simulink model "extended_estimator"  (R2022b)
settings: Solver=FixedStepAuto  StartTime=0.0  StopTime=30  FixedStep=0.001  RelTol=1e-3
values from neighbouring files (symbols this model uses):
  A = -3    [para.m]
  As = [0 1 0;-omega^2 0 0; 1 0 -3]    [para.m]
  B = 1    [para.m]
  Bs = [0 ; 0 ;1]    [para.m]
  C = 1    [para.m]
  Cs = [0 0 1]    [para.m]
  D = 0    [para.m]
  Ds = 0    [para.m]
  K = place(A,B,-5)    [para.m]
  L = place(As',Cs',[-19 -20 -21])'    [para.m]
  omega = 10    [para.m]
settings Model: Creator=mxiaoxin  LastModifiedBy=mxiaoxin

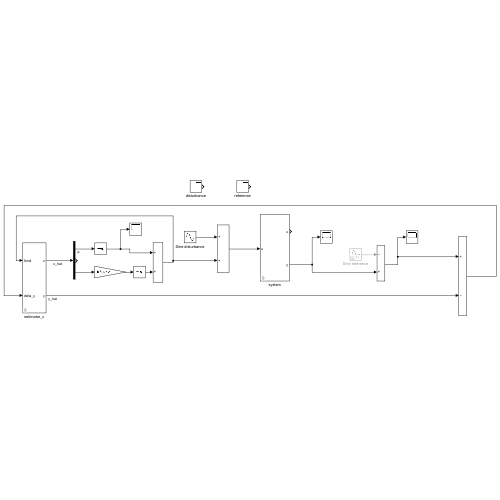
[thumbnail: Simulink's stored preview of the top-level diagram]
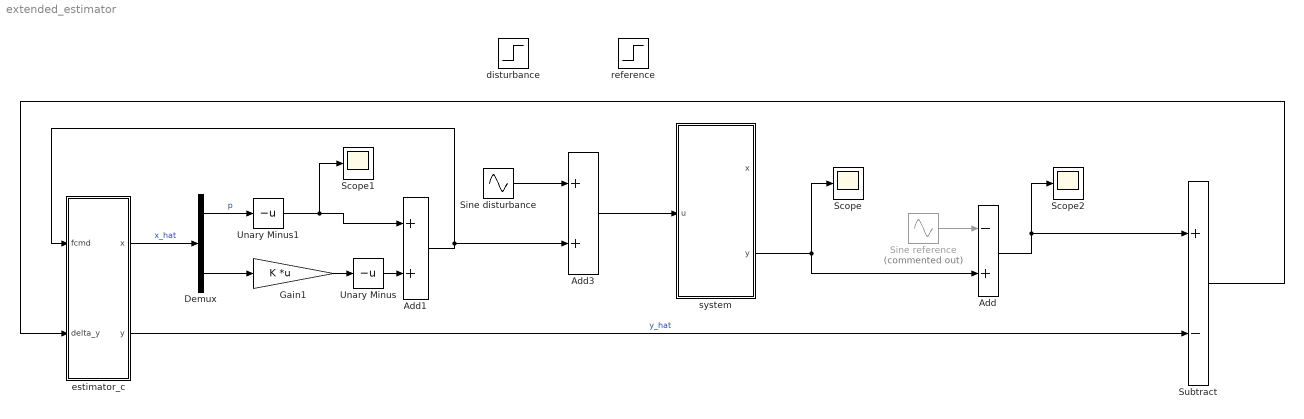
== system extended_estimator ==
  Add : Sum  Inputs=-+
  Add1 : Sum
  Add3 : Sum
  Demux : Demux  Outputs=3
  Gain1 : Gain  Gain=K  Multiplication=Matrix(K*u) (u vector)
  Scope : Scope
  Scope1 : Scope
  Scope2 : Scope
  Sine disturbance : Sin  Frequency=omega  Phase=180  SampleTime=0
  Sine reference : Sin  Commented=on  Frequency=omega  SampleTime=0
  Subtract : Sum  Inputs=+-
  Unary Minus : UnaryMinus
  Unary Minus1 : UnaryMinus
  disturbance : Step  SampleTime=0
  estimator_c : Subsystem  mask{x_A=As, x_B=Bs, x_C=Cs, x_D=Ds, xl=L}
      mask prompts: x_A "A"; x_B "B"; x_C "C"; x_D "D"; xl "L"
      mask DialogControl ParameterGroupVar Prompt: 系统
      mask DialogControl Container3 Prompt: feedback
  reference : Step  Time=0  SampleTime=0
  system : Subsystem  mask{Ac=A, Bc=B, Cc=C, Dc=D, x_0=0}
      mask DialogControl ParameterGroupVar Prompt: 参数
  wires:
  Subtract/1 -> estimator_c/2(delta_y)
  estimator_c/1(x) -> Demux/1  "x_hat"
  Unary Minus1/1 -> Add1/1, Scope1/1
  Gain1/1 -> Unary Minus/1
  Unary Minus/1 -> Add1/2
  Demux/1 -> Unary Minus1/1  "p"
  system/2(y) -> Add/2, Scope/1
  Add1/1 -> Add3/2, estimator_c/1(fcmd)
  Add3/1 -> system/1(u)
  estimator_c/2(y) -> Subtract/2  "y_hat"
  Sine disturbance/1 -> Add3/1
  Demux/3 -> Gain1/1
  Add/1 -> Subtract/1, Scope2/1
  Sine reference/1 -> Add/1

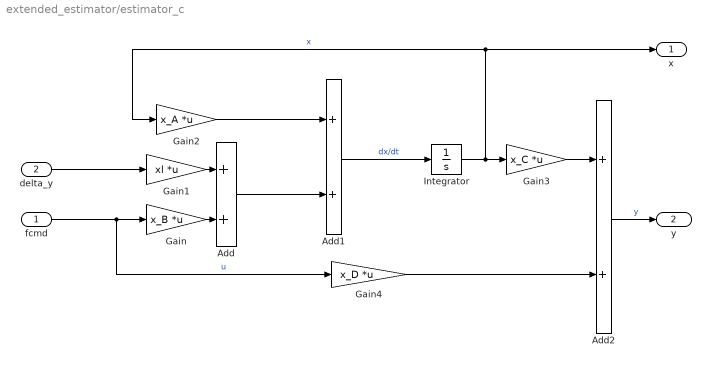
== system extended_estimator/estimator_c ==
  fcmd : Inport
  delta_y : Inport  Port=2
  Add : Sum
  Add1 : Sum
  Add2 : Sum
  Gain : Gain  Gain=x_B  Multiplication=Matrix(K*u)
  Gain1 : Gain  Gain=xl  Multiplication=Matrix(K*u)
  Gain2 : Gain  Gain=x_A  Multiplication=Matrix(K*u)
  Gain3 : Gain  Gain=x_C  Multiplication=Matrix(K*u)
  Gain4 : Gain  Gain=x_D  Multiplication=Matrix(K*u)
  Integrator : Integrator
  x : Outport
  y : Outport  Port=2
  wires:
  Gain2/1 -> Add1/1
  Add/1 -> Add1/2
  Add1/1 -> Integrator/1  "dx/dt"
  Integrator/1 -> Gain3/1, x/1, Gain2/1  "x"
  Gain1/1 -> Add/1
  delta_y/1 -> Gain1/1
  fcmd/1 -> Gain/1, Gain4/1  "u"
  Gain/1 -> Add/2
  Gain3/1 -> Add2/1
  Gain4/1 -> Add2/2
  Add2/1 -> y/1  "y"

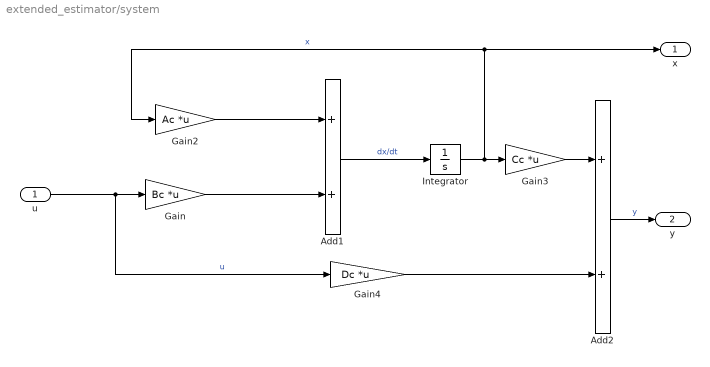
== system extended_estimator/system ==
  u : Inport
  Add1 : Sum
  Add2 : Sum
  Gain : Gain  Gain=Bc  Multiplication=Matrix(K*u)
  Gain2 : Gain  Gain=Ac  Multiplication=Matrix(K*u)
  Gain3 : Gain  Gain=Cc  Multiplication=Matrix(K*u)
  Gain4 : Gain  Gain=Dc  Multiplication=Matrix(K*u)
  Integrator : Integrator  InitialCondition=x_0
  x : Outport
  y : Outport  Port=2
  wires:
  Gain2/1 -> Add1/1
  Gain/1 -> Add1/2
  Add1/1 -> Integrator/1  "dx/dt"
  Integrator/1 -> Gain3/1, Gain2/1, x/1  "x"
  u/1 -> Gain/1, Gain4/1  "u"
  Gain3/1 -> Add2/1
  Gain4/1 -> Add2/2
  Add2/1 -> y/1  "y"
